simulink model "DiscreteIntegrator_TestGen12"  (R2017b)
settings: Solver=FixedStepDiscrete  StartTime=0.0  StopTime=10.0  RelTol=1e-3
undefined symbols (not defined in the file): Block_TestLib, DiscIntNeverNeededParam, enable_trigger
settings Model: Creator=hbourbou  LastModifiedBy=hbourbou
settings DebuggingCC: ParameterOverflowMsg=none

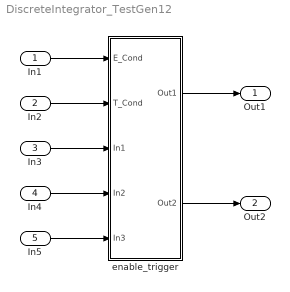
== system DiscreteIntegrator_TestGen12 ==
  In1 : Inport
  In2 : Inport  Port=2
  In3 : Inport  Port=3
  In4 : Inport  Port=4
  In5 : Inport  Port=5
  enable_trigger : Subsystem  AncestorBlock=Block_TestLib/enable_trigger
  Out1 : Outport
  Out2 : Outport  Port=2
  wires:
  In1/1 -> enable_trigger/1(E_Cond)
  In2/1 -> enable_trigger/2(T_Cond)
  In3/1 -> enable_trigger/3(In1)
  In4/1 -> enable_trigger/4(In2)
  In5/1 -> enable_trigger/5(In3)
  enable_trigger/1(Out1) -> Out1/1
  enable_trigger/2(Out2) -> Out2/1

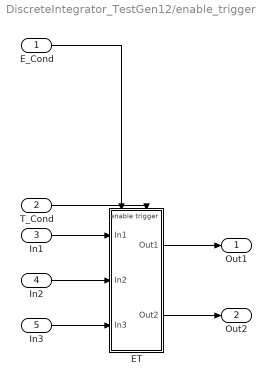
== system DiscreteIntegrator_TestGen12/enable_trigger ==
  E_Cond : Inport  OutDataTypeStr=boolean
  T_Cond : Inport  Port=2  OutDataTypeStr=boolean
  In1 : Inport  Port=3
  In2 : Inport  Port=4
  In3 : Inport  Port=5
  ET : Subsystem  TreatAsAtomicUnit=on
  Out1 : Outport
  Out2 : Outport  Port=2
  wires:
  T_Cond/1 -> ET/Trigger
  E_Cond/1 -> ET/Enable
  In1/1 -> ET/1(In1)
  In2/1 -> ET/2(In2)
  In3/1 -> ET/3(In3)
  ET/1(Out1) -> Out1/1
  ET/2(Out2) -> Out2/1

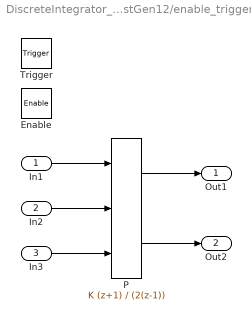
== system DiscreteIntegrator_TestGen12/enable_trigger/ET ==
  In1 : Inport  OutDataTypeStr=int8  PortDimensions=1
  In2 : Inport  Port=2
  In3 : Inport  Port=3
  Enable : EnablePort
  Trigger : TriggerPort  VariantControl=Variant
  P : DiscreteIntegrator  IntegratorMethod=Accumulation: Trapezoidal  gainval=2.0  ExternalReset=rising  InitialConditionSource=external  InitialCondition=7  SampleTime=-1  OutDataTypeStr=int16  RndMeth=Round  SaturateOnIntegerOverflow=on  LimitOutput=on  UpperSaturationLimit=100  LowerSaturationLimit=5  ShowSaturationPort=on  ICPrevOutput=DiscIntNeverNeededParam  ICPrevScaledInput=DiscIntNeverNeededParam
  Out1 : Outport
  Out2 : Outport  Port=2
  wires:
  In1/1 -> P/1
  In2/1 -> P/2
  In3/1 -> P/3
  P/1 -> Out1/1
  P/2 -> Out2/1
